simulink model "OneRobot_Sliding"  (R2014b)
settings: Solver=ode45  StartTime=0.3  StopTime=10  FixedStep=0.01  RelTol=1e-3
settings Model: Creator=mshahria  LastModifiedBy=mshahria

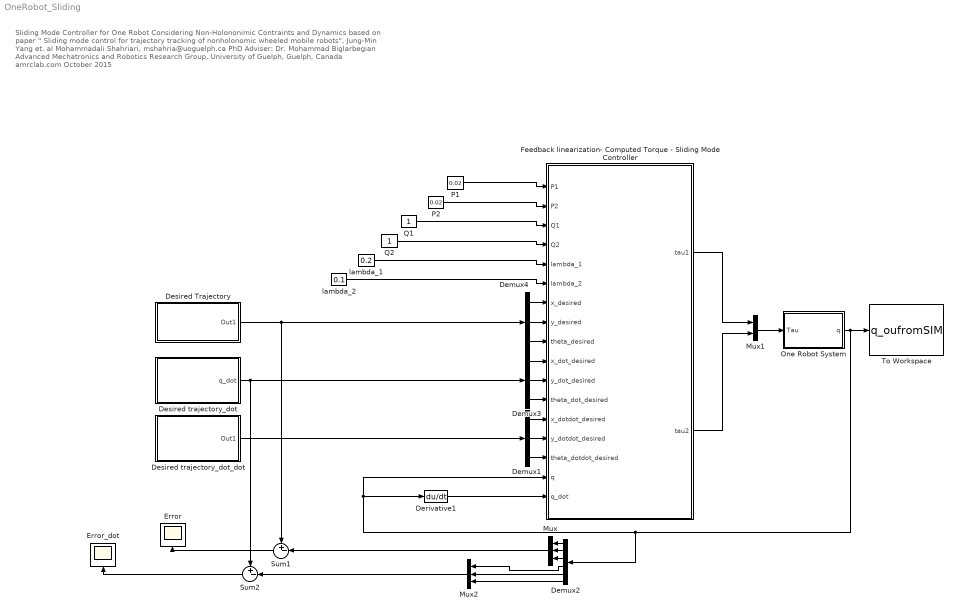
== system OneRobot_Sliding ==
  note: Sliding Mode Controller for One Robot Considering Non-Holononimic Contraints and Dynamics
      | based on paper " Sliding mode control for trajectory tracking of nonholonomic wheeled mobile robots", Jung-Min Yang et. al
      | Mohammadali Shahriari, mshahria@uoguelph.ca
      | PhD Adviser: Dr. Mohammad Biglarbegian
      | Advanced Mechatronics and Robotics Research Group,
      | University of Guelph,
      | Guelph, Canada
      | amrclab.com
      | October 2015
  " One Robot System" : Subsystem
  Demux1 : Demux  Outputs=3
  Demux2 : Demux  Outputs=6
  Demux3 : Demux  Outputs=3
  Demux4 : Demux  Outputs=3
  Derivative1 : Derivative
  Desired Trajectory : Subsystem
  Desired trajectory_dot : Subsystem
  Desired trajectory_dot_dot : Subsystem
  Error : Scope
      settings: SaveName=ScopeData2
  Error_dot : Scope
  "Feedback linearization- Computed Torque - Sliding Mode Controller " : MATLAB Function  TreatAsAtomicUnit=on
  Mux : Mux  Inputs=3
  Mux1 : Mux  Inputs=2
  Mux2 : Mux  Inputs=3
  P1 : Constant  Value=0.02
  P2 : Constant  Value=0.02
  Q1 : Constant
  Q2 : Constant
  Sum1 : Sum  Inputs=+-|
  Sum2 : Sum  Inputs=+-|
  To Workspace : ToWorkspace  VariableName=q_oufromSIM  SampleTime=-1
  "lambda_1 " : Constant  Value=0.2
  lambda_2 : Constant  Value=0.1
  wires:
  " One Robot System"/1(q) -> "Feedback linearization- Computed Torque - Sliding Mode Controller "/16(q), Derivative1/1, Demux2/1, To Workspace/1
  Derivative1/1 -> "Feedback linearization- Computed Torque - Sliding Mode Controller "/17(q_dot)
  "Feedback linearization- Computed Torque - Sliding Mode Controller "/1(tau1) -> Mux1/1
  "Feedback linearization- Computed Torque - Sliding Mode Controller "/2(tau2) -> Mux1/2
  Mux1/1 -> " One Robot System"/1(Tau)
  Demux1/3 -> "Feedback linearization- Computed Torque - Sliding Mode Controller "/15(theta_dotdot_desired)
  Demux1/2 -> "Feedback linearization- Computed Torque - Sliding Mode Controller "/14(y_dotdot_desired)
  Demux1/1 -> "Feedback linearization- Computed Torque - Sliding Mode Controller "/13(x_dotdot_desired)
  Demux2/1 -> Mux/1
  Demux2/2 -> Mux/2
  Demux2/3 -> Mux/3
  "lambda_1 "/1 -> "Feedback linearization- Computed Torque - Sliding Mode Controller "/5(lambda_1)
  lambda_2/1 -> "Feedback linearization- Computed Torque - Sliding Mode Controller "/6(lambda_2)
  Desired trajectory_dot_dot/1(Out1) -> Demux1/1
  Desired Trajectory/1(Out1) -> Demux4/1, Sum1/1
  Desired trajectory_dot/1(q_dot) -> Demux3/1, Sum2/1
  Q2/1 -> "Feedback linearization- Computed Torque - Sliding Mode Controller "/4(Q2)
  Q1/1 -> "Feedback linearization- Computed Torque - Sliding Mode Controller "/3(Q1)
  P2/1 -> "Feedback linearization- Computed Torque - Sliding Mode Controller "/2(P2)
  P1/1 -> "Feedback linearization- Computed Torque - Sliding Mode Controller "/1(P1)
  Demux4/3 -> "Feedback linearization- Computed Torque - Sliding Mode Controller "/9(theta_desired)
  Demux3/3 -> "Feedback linearization- Computed Torque - Sliding Mode Controller "/12(theta_dot_desired)
  Demux4/1 -> "Feedback linearization- Computed Torque - Sliding Mode Controller "/7(x_desired)
  Demux4/2 -> "Feedback linearization- Computed Torque - Sliding Mode Controller "/8(y_desired)
  Demux3/2 -> "Feedback linearization- Computed Torque - Sliding Mode Controller "/11(y_dot_desired)
  Demux3/1 -> "Feedback linearization- Computed Torque - Sliding Mode Controller "/10(x_dot_desired)
  Mux/1 -> Sum1/2
  Mux2/1 -> Sum2/2
  Demux2/6 -> Mux2/3
  Demux2/5 -> Mux2/2
  Demux2/4 -> Mux2/1
  Sum1/1 -> Error/1
  Sum2/1 -> Error_dot/1

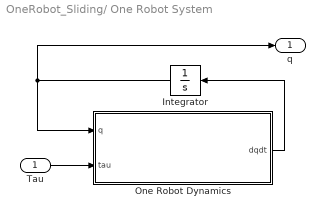
== system OneRobot_Sliding/ One Robot System ==
  Tau : Inport
  Integrator : Integrator  InitialCondition=|  LimitOutput=on  UpperSaturationLimit=[inf,inf,inf,0.4,0.4,0.5]  LowerSaturationLimit=[-inf,-inf,-inf,-0.4,-0.4,-0.5]
      | [.2136; 0.7015
      | ;pi/3;0;0;0]
  One Robot Dynamics : MATLAB Function  TreatAsAtomicUnit=on
  q : Outport
  wires:
  Integrator/1 -> q/1, One Robot Dynamics/1(q)
  One Robot Dynamics/1(dqdt) -> Integrator/1
  Tau/1 -> One Robot Dynamics/2(tau)

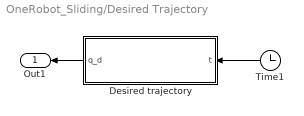
== system OneRobot_Sliding/Desired Trajectory ==
  Desired trajectory : MATLAB Function  TreatAsAtomicUnit=on
  Time1 : Clock
  Out1 : Outport
  wires:
  Time1/1 -> Desired trajectory/1(t)
  Desired trajectory/1(q_d) -> Out1/1

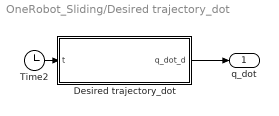
== system OneRobot_Sliding/Desired trajectory_dot ==
  Desired trajectory_dot : MATLAB Function  TreatAsAtomicUnit=on
  Time2 : Clock
  q_dot : Outport
  wires:
  Desired trajectory_dot/1(q_dot_d) -> q_dot/1
  Time2/1 -> Desired trajectory_dot/1(t)

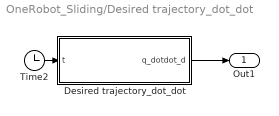
== system OneRobot_Sliding/Desired trajectory_dot_dot ==
  Desired trajectory_dot_dot : MATLAB Function  TreatAsAtomicUnit=on
  Time2 : Clock
  Out1 : Outport
  wires:
  Time2/1 -> Desired trajectory_dot_dot/1(t)
  Desired trajectory_dot_dot/1(q_dotdot_d) -> Out1/1

== matlab function OneRobot_Sliding/Desired Trajectory/Desired trajectory ==
  data: t input; q_d output
function q_d = fcn(t)

q_d = q_desired(t);

== matlab function OneRobot_Sliding/ One Robot System/One Robot Dynamics ==
  data: dqdt output; q input; tau input
function dqdt= Robot_ode(q,tau)
dqdt=zeros(6,1);
% global tau_l tau_r; 
tau_l=tau(1);
tau_r=tau(2);

x_dot=q(4);
y_dot=q(5);
theta=q(3);
theta_dot=q(6);
q_dotdot = Qdotdot(tau_l,tau_r,theta,theta_dot,x_dot,y_dot);

dqdt(1)=q(4);
dqdt(2)=q(5);
dqdt(3)=q(6);
dqdt(4)=(q_dotdot(1));
dqdt(5)=(q_dotdot(2));
dqdt(6)=(q_dotdot(3));

== matlab function OneRobot_Sliding/Feedback linearization- Computed Torque - Sliding Mode Controller  ==
  data: P1 input; P2 input; Q1 input; Q2 input; lambda_1 input; lambda_2 input; x_desired input; y_desired input; theta_desired input; x_dot_desired input; y_dot_desired input; theta_dot_desired input; x_dotdot_desired input; y_dotdot_desired input; theta_dotdot_desired input; tau1 output; q input; q_dot input; tau2 output
function [tau1,tau2]= controller(P1,P2,Q1,Q2,lambda_1,lambda_2,x_desired,y_desired,theta_desired,x_dot_desired,y_dot_desired,theta_dot_desired, x_dotdot_desired, y_dotdot_desired,theta_dotdot_desired,q,q_dot)

theta=q(3);
theta_dot=q(6);
x_dotdot=q_dot(4);
y_dotdot=q_dot(5);
theta_dotdot=q_dot(6);
x=q(1);
y=q(2);
x_dot=q(4);
y_dot=q(5);
vc=sqrt(x_dot^2+y_dot^2);

u=U_sliding(P1,P2,Q1,Q2,lambda_1,lambda_2,theta,theta_dot,theta_desired,theta_dot_desired,x,x_dot,x_desired,x_dot_desired,x_dotdot_desired,y,y_dot,y_desired,y_dot_desired,y_dotdot_desired);

Tau= Tau_fdbckln(theta,theta_dot,theta_dotdot_desired,x_dot,x_dotdot_desired,y_dot,y_dotdot_desired)+ Hqfun(theta)*u;
tau1=Tau(1);
tau2=Tau(2);

== matlab function OneRobot_Sliding/Desired trajectory_dot_dot/Desired trajectory_dot_dot ==
  data: t input; q_dotdot_d output
function q_dotdot_d = fcn(t)

q_dotdot_d = q_dotdot_desired(t);

== matlab function OneRobot_Sliding/Desired trajectory_dot/Desired trajectory_dot ==
  data: t input; q_dot_d output
function q_dot_d = fcn(t)

q_dot_d = q_dot_desired(t);
